simulink model "noise"  (R2023b)
settings: Solver=VariableStepAuto  StartTime=0.0  StopTime=10.0  RelTol=1e-3
settings Model: Creator=ASUS  LastModifiedBy=ASUS

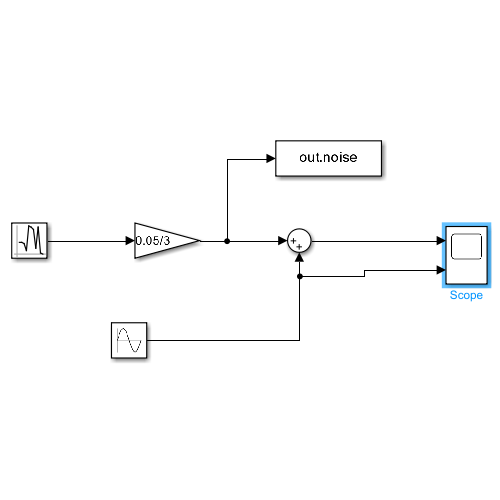
[thumbnail: Simulink's stored preview of the top-level diagram]
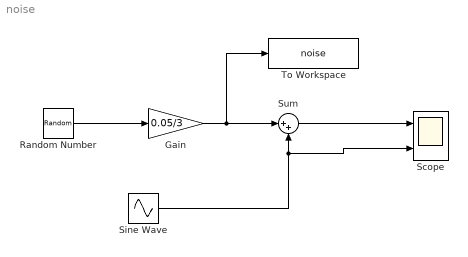
== system noise ==
  Gain : Gain  Gain=0.05/3
  Random Number : RandomNumber  SampleTime=1e-3
  Scope : Scope  NumInputPorts=2
  Sine Wave : Sin  Amplitude=0.5  Frequency=6.28  SampleTime=0
  Sum : Sum  Inputs=|++
  To Workspace : ToWorkspace  VariableName=noise  SaveFormat=Timeseries  SampleTime=-1
  wires:
  Sine Wave/1 -> Sum/2, Scope/2
  Sum/1 -> Scope/1
  Random Number/1 -> Gain/1
  Gain/1 -> Sum/1, To Workspace/1
